simulink model "Ex_14_Luenberger_Observer"  (Simulink 9.0)
settings: Solver=VariableStepAuto  StartTime=0.0  StopTime=t_max  FixedStep=jointObj.Ts/10  RelTol=1e-3
values from neighbouring files (symbols this model uses):
  t_max = f_max    (= 100)    [Ex_00_example_config.m]
undefined symbols (not defined in the file or in its folder): C, Cc
undefined symbols (not defined in the file): jointObj
libraries: simulink x1, cjt_library_models x1, cstblocks x1
settings Model: Creator=joern  LastModifiedBy=J�rn
settings DebuggingCC: UnderspecifiedInitializationDetection=Simplified  MergeDetectMultiDrivingBlocksExec=error  SolverPrmCheckMsg=warning
settings GRTTargetCC: GeneratePreprocessorConditionals=Disable all
settings ConfigComp: CovSFcnEnable=off

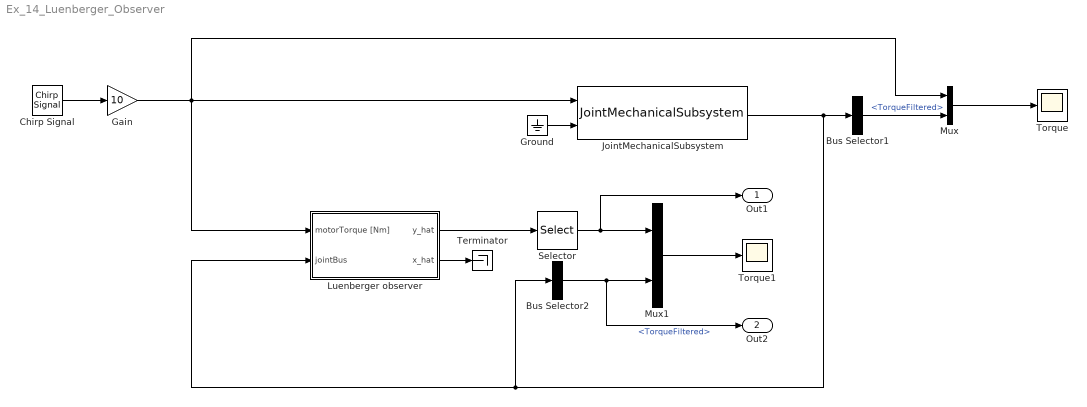
== system Ex_14_Luenberger_Observer ==
  Bus Selector1 : BusSelector  OutputSignals=TorqueFiltered
  Bus Selector2 : BusSelector  OutputSignals=TorqueFiltered
  Chirp Signal : simulink/Sources/Chirp Signal  f1=f_min  T=t_max  f2=f_max
  Gain : Gain  Gain=10
  Ground : Ground
  JointMechanicalSubsystem : cjt_library_models/Joint models/JointMechanicalSubsystem  jointObj=jointObj  fc_vel=1000  fc_torque=1000  input_delay=1  output_delay=1  quantize=on  quantize_bits=19  input_noise_enabled=on  output_noise_enabled=on  var_u=0.12^2  var_y=1.8e-10
  Luenberger observer : Subsystem  AncestorBlock=cjt_library_observers/Observers/Luenberger observer  mask(Luenberger observer){jointObj=jointObj, outputIdx=[1 7], poles=2*pi*[-60 -70 -80]}
      mask prompts: jointObj "Joint Object"; outputIdx "Measured outputs (indices)"; poles "Observer poles"
      mask help:
      | This block implements a standard Luenberger state estimator based on a linear state-space model of the joint. Therefore, the block relies on the function 'place' shipped with the Mathworks Control System Toolbox (required dependency for this block).
      |
      | Click >Help< for further documentation.
      mask init:
      | mask_Luenberger_observer
      mask Help:
      | This block implements a standard Luenberger state estimator based on a linear state-space model of the joint. Therefore, the block relies on the function 'place' shipped with the Mathworks Control System Toolbox (required dependency for this block).
      | 
      | <b>Mask parameters</b>
      | <b>Joint Object</b>: The class name of the CJT joint class name or the variable representing an instance of a CJT joint class.
      | <b>Measurement Outputs</b>: vector of indices defining the elements of the output vector to be used for observation. Choices are
      | 1 - motor angle
      | 2 - gear angle
      | 3 - link  angle
      | 4 - motor velocity
      | 5 - gear velocity
      | 6  - link velocity
      | 7  - spring torque
      | 
      | <b>Observer poles</b>: Where to place the poles of the state observer. All poles need to be supplied, i.e. the same number as rows in the A state-space matrix of the chosen actuator model.
      | 
      | <b>References</b>
      | [1] Franklin, G.F., J.D. Powell, and M.L. Workman, Digital Control of Dynamic Systems, Second Edition, Addison-Wesley, 1990.
      | 
      | [2] Lewis, F., Optimal Estimation, John Wiley & Sons, Inc, 1986.
  Mux : Mux  Inputs=2
  Mux1 : Mux  Inputs=2
  Selector : Selector  InputPortWidth=2  IndexOptions=Index vector (dialog)  Indices=[2]  OutputSizes=1
  Terminator : Terminator
  Torque : Scope
  Torque1 : Scope
  Out1 : Outport
  Out2 : Outport  Port=2
  wires:
  Mux/1 -> Torque/1
  Ground/1 -> JointMechanicalSubsystem/2
  JointMechanicalSubsystem/1 -> Luenberger observer/2(jointBus), Bus Selector2/1, Bus Selector1/1
  Gain/1 -> Luenberger observer/1(motorTorque [Nm]), JointMechanicalSubsystem/1, Mux/1
  Chirp Signal/1 -> Gain/1
  Bus Selector1/1 -> Mux/2  "<TorqueFiltered>"
  Luenberger observer/1(y_hat) -> Selector/1
  Bus Selector2/1 -> Out2/1, Mux1/2  "<TorqueFiltered>"
  Selector/1 -> Out1/1, Mux1/1
  Mux1/1 -> Torque1/1
  Luenberger observer/2(x_hat) -> Terminator/1

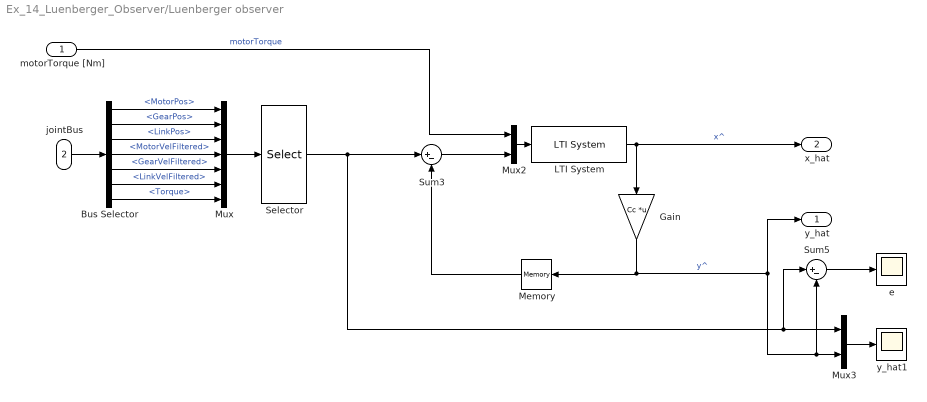
== system Ex_14_Luenberger_Observer/Luenberger observer ==
  motorTorque [Nm] : Inport
  jointBus : Inport  Port=2
  Bus Selector : BusSelector  OutputSignals=MotorPos,GearPos,LinkPos,MotorVelFiltered,GearVelFiltered,LinkVelFiltered,Torque
  Gain : Gain  Gain=Cc  Multiplication=Matrix(K*u)
  LTI System : cstblocks/LTI System  sys=sys_hat_tust  IC=[]
  Memory : Memory  LinearizeMemory=on  LinearizeAsDelay=on
  Mux : Mux  Inputs=7
  Mux2 : Mux  Inputs=2
  Mux3 : Mux  Inputs=2
  Selector : Selector  InputPortWidth=size(C,1)  IndexOptions=Index vector (dialog)  Indices=outputIdx  OutputSizes=1
  Sum3 : Sum  Inputs=|+-
  Sum5 : Sum  Inputs=|+-
  e : Scope
  y_hat1 : Scope
  y_hat : Outport
  x_hat : Outport  Port=2
  wires:
  Mux/1 -> Selector/1
  Bus Selector/1 -> Mux/1  "<MotorPos>"
  Bus Selector/5 -> Mux/5  "<GearVelFiltered>"
  Bus Selector/3 -> Mux/3  "<LinkPos>"
  Bus Selector/6 -> Mux/6  "<LinkVelFiltered>"
  Bus Selector/2 -> Mux/2  "<GearPos>"
  Bus Selector/4 -> Mux/4  "<MotorVelFiltered>"
  jointBus/1 -> Bus Selector/1
  Bus Selector/7 -> Mux/7  "<Torque>"
  Gain/1 -> Memory/1, Mux3/2, Sum5/2, y_hat/1  "y^"
  Sum3/1 -> Mux2/2
  Selector/1 -> Sum5/1, Mux3/1, Sum3/1
  Mux2/1 -> LTI System/1
  LTI System/1 -> x_hat/1, Gain/1  "x^"
  motorTorque [Nm]/1 -> Mux2/1  "motorTorque"
  Sum5/1 -> e/1
  Mux3/1 -> y_hat1/1
  Memory/1 -> Sum3/2
